simulink model "Two_wheeled_RobotModel_UsingSimulink"  (R2020a)
settings: Solver=VariableStepAuto  StartTime=0.0  StopTime=10.0  RelTol=1e-3
values from neighbouring files (symbols this model uses):
  d = 0.045    [params_sliding.m]
  g = 9.81    [params_sliding.m]
  I3 = 0.003483    [params_sliding.m]
  mc = 0.3    [params_sliding.m]
  ms = 5.16    [params_sliding.m]
  R = 0.065    [params_sliding.m]
settings Model: Creator=User  LastModifiedBy=User

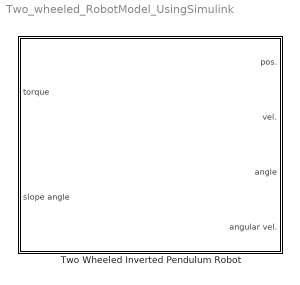
== system Two_wheeled_RobotModel_UsingSimulink ==
  Two Wheeled Inverted Pendulum Robot : Subsystem

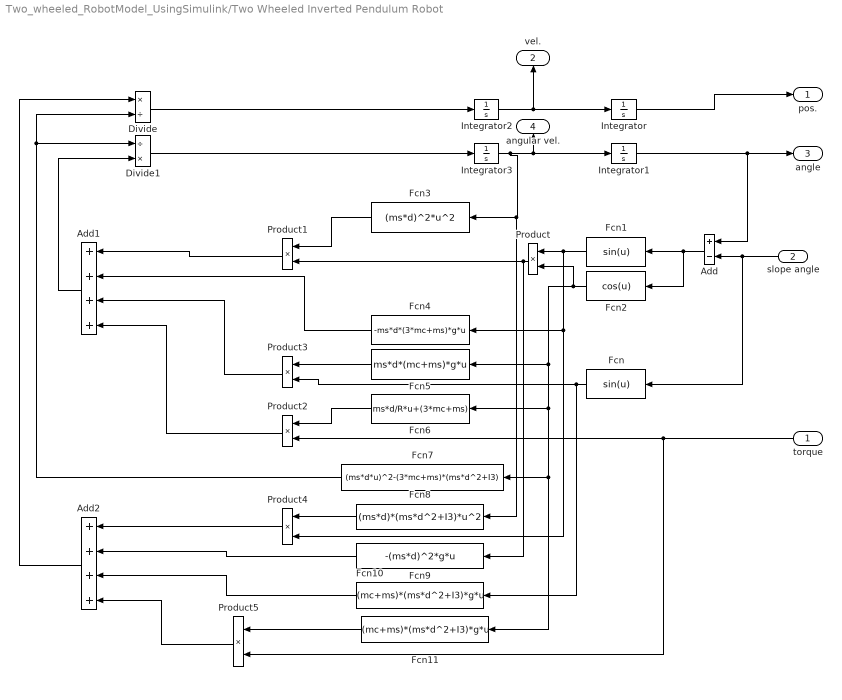
== system Two_wheeled_RobotModel_UsingSimulink/Two Wheeled Inverted Pendulum Robot ==
  torque : Inport
  slope angle : Inport  Port=2
  Add : Sum  Inputs=+-
  Add1 : Sum  Inputs=++++
  Add2 : Sum  Inputs=++++
  Divide : Product  Inputs=*/
  Divide1 : Product  Inputs=/*
  Fcn : Fcn  Expr=sin(u)
  Fcn1 : Fcn  Expr=sin(u)
  Fcn10 : Fcn  Expr=(mc+ms)*(ms*d^2+I3)*g*u
  Fcn11 : Fcn  Expr=(mc+ms)*(ms*d^2+I3)*g*u
  Fcn2 : Fcn  Expr=cos(u)
  Fcn3 : Fcn  Expr=(ms*d)^2*u^2
  Fcn4 : Fcn  Expr=-ms*d*(3*mc+ms)*g*u
  Fcn5 : Fcn  Expr=ms*d*(mc+ms)*g*u
  Fcn6 : Fcn  Expr=ms*d/R*u+(3*mc+ms)
  Fcn7 : Fcn  Expr=(ms*d*u)^2-(3*mc+ms)*(ms*d^2+I3)
  Fcn8 : Fcn  Expr=(ms*d)*(ms*d^2+I3)*u^2
  Fcn9 : Fcn  Expr=-(ms*d)^2*g*u
  Integrator{,1..3} (4 alike) : Integrator
  Product{,1..5} (6 alike) : Product
  pos. : Outport
  vel. : Outport  Port=2
  angle : Outport  Port=3
  angular vel. : Outport  Port=4
  wires:
  Product4/1 -> Add2/1
  Integrator1/1 -> angle/1, Add/1
  Add/1 -> Fcn2/1, Fcn1/1
  Add1/1 -> Divide1/2
  Integrator3/1 -> Fcn3/1, Fcn8/1, angular vel./1, Integrator1/1
  Divide/1 -> Integrator2/1
  Integrator2/1 -> vel./1, Integrator/1
  Product3/1 -> Add1/3
  Fcn/1 -> Fcn10/1, Product3/2
  Integrator/1 -> pos./1
  Product1/1 -> Add1/1
  Fcn6/1 -> Product2/1
  Fcn1/1 -> Fcn4/1, Product4/2, Product/1
  slope angle/1 -> Fcn/1, Add/2
  torque/1 -> Product2/2, Product5/2
  Fcn7/1 -> Divide/2, Divide1/1
  Fcn2/1 -> Fcn11/1, Fcn7/1, Fcn6/1, Fcn5/1, Product/2
  Product/1 -> Product1/2, Fcn9/1
  Fcn5/1 -> Product3/1
  Divide1/1 -> Integrator3/1
  Product2/1 -> Add1/4
  Fcn3/1 -> Product1/1
  Fcn4/1 -> Add1/2
  Product5/1 -> Add2/4
  Fcn10/1 -> Add2/3
  Fcn8/1 -> Product4/1
  Fcn9/1 -> Add2/2
  Add2/1 -> Divide/1
  Fcn11/1 -> Product5/1
